simulink model "Factorial2016"  (R2016a)
settings: Solver=FixedStepDiscrete  StartTime=0.0  StopTime=10.0  RelTol=1e-3
settings Model: Creator=pc  LastModifiedBy=pc
settings OptimizationCC: DefaultParameterBehavior=Inlined  OptimizeModelRefInitCode=on  LifeSpan=1
settings SFSimCC: SimCustomHeaderCode=|
  | #include "Led.h"
  | #include "switch.h"
settings SFSimCC: SimUserSources=|
  | Led.c
  | switch.c
settings RTWCC: SystemTargetFile=ert.tlc  GenCodeOnly=on  GenerateMakefile=off  TemplateMakefile=ert_default_tmf  GenerateReport=on  IncludeHyperlinkInReport=on  LaunchReport=on  GenerateTraceInfo=on  GenerateTraceReport=on  GenerateTraceReportSl=on  GenerateTraceReportSf=on  GenerateTraceReportEml=on
settings CodeAppCC: ForceParamTrailComments=on  IgnoreCustomStorageClasses=off  OperatorAnnotations=on  SimulinkDataObjDesc=on  SFDataObjDesc=on  MATLABFcnDesc=on  InsertBlockDesc=on  MATLABSourceComments=on
settings ERTTargetCC: GenerateSampleERTMain=on  SuppressErrorStatus=on  InlinedParameterPlacement=NonHierarchical  ERTCustomFileTemplate=example_file_process.tlc  EnableUserReplacementTypes=on

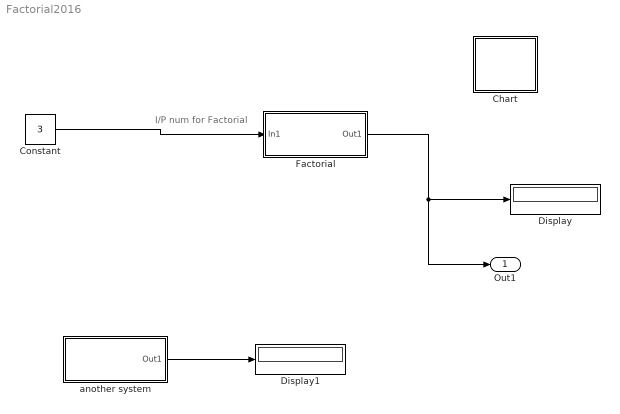
== system Factorial2016 ==
  note: I/P num for Factorial
  Chart : Stateflow chart  TreatAsAtomicUnit=on
  Constant : Constant  Value=3  OutDataTypeStr=int32  SampleTime=-1
  Display : Display
  Display1 : Display
  Factorial : Subsystem  TreatAsAtomicUnit=on
  another system : Subsystem  TreatAsAtomicUnit=on
  Out1 : Outport  OutDataTypeStr=int32
  wires:
  Factorial/1(Out1) -> Display/1, Out1/1
  Constant/1 -> Factorial/1(In1)
  another system/1(Out1) -> Display1/1

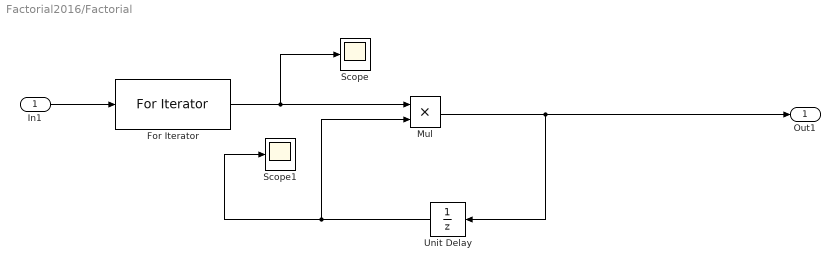
== system Factorial2016/Factorial ==
  In1 : Inport  OutDataTypeStr=int32
  For Iterator : ForIterator  ResetStates=reset  IterationSource=external
  Mul : Product  OutDataTypeStr=Inherit: Same as first input
  Scope : Scope
  Scope1 : Scope
  Unit Delay : UnitDelay  InitialCondition=1  SampleTime=-1
  Out1 : Outport  OutDataTypeStr=int32
  wires:
  In1/1 -> For Iterator/1
  For Iterator/1 -> Scope/1, Mul/1
  Mul/1 -> Unit Delay/1, Out1/1
  Unit Delay/1 -> Scope1/1, Mul/2

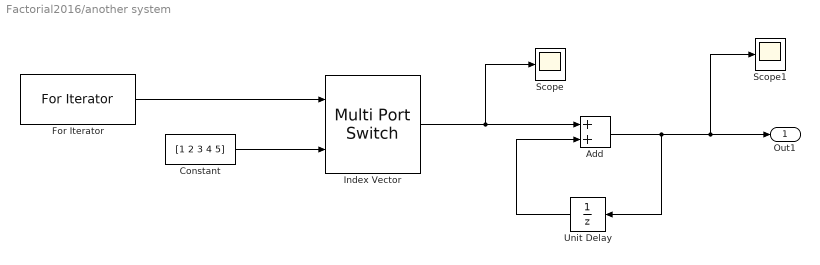
== system Factorial2016/another system ==
  Add : Sum
  Constant : Constant  Value=[1 2 3 4 5]
  For Iterator : ForIterator  ResetStates=reset  IndexMode=Zero-based
  Index Vector : MultiPortSwitch  DataPortOrder=Zero-based contiguous  Inputs=1  zeroidx=on
  Scope : Scope
  Scope1 : Scope
  Unit Delay : UnitDelay  SampleTime=-1
  Out1 : Outport
  wires:
  For Iterator/1 -> Index Vector/1
  Constant/1 -> Index Vector/2
  Index Vector/1 -> Scope/1, Add/1
  Unit Delay/1 -> Add/2
  Add/1 -> Unit Delay/1, Scope1/1, Out1/1

== stateflow chart Factorial2016/Chart ==
  (default) -> (junction 2) : {Led_TurnOn(LED_ID_1);}
  data: LED_ID_1 parameter uint16
